simulink model "ABLS_Model"  (R2025a)
settings: Solver=FixedStepDiscrete  StartTime=0.0  StopTime=10.0  FixedStep=0.01  RelTol=1e-3
undefined symbols (not defined in the file): dspblkCoreblockFVToolHelper, gcbh, Ts
libraries: simulink x3
settings Model: Creator=Gagan  LastModifiedBy=Gagan

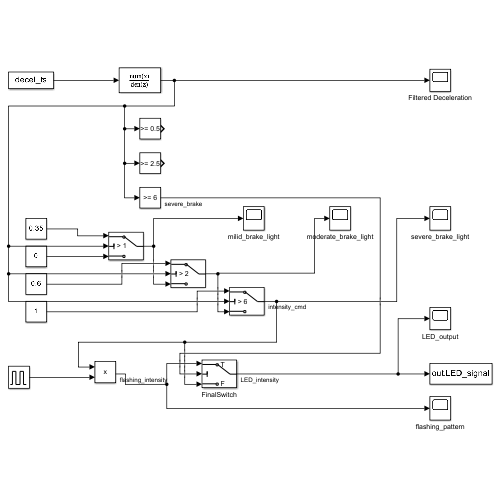
[thumbnail: Simulink's stored preview of the top-level diagram]
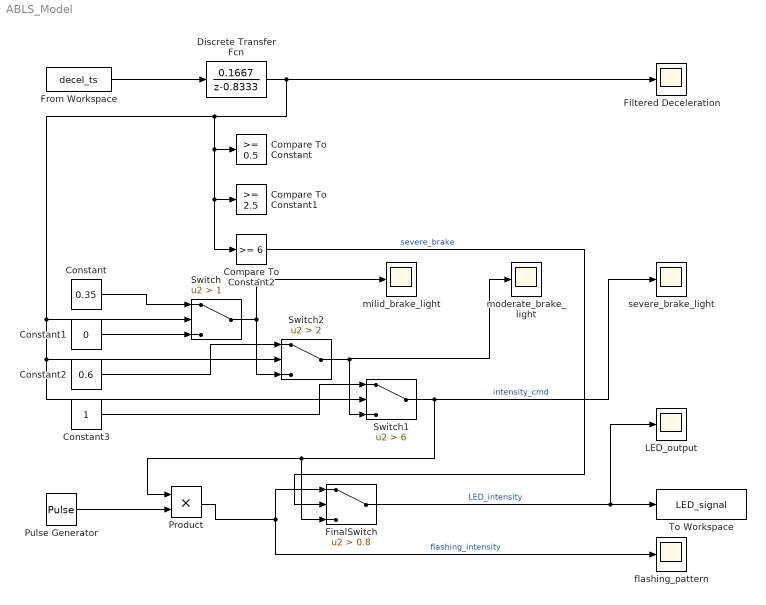
== system ABLS_Model ==
  Compare To Constant : simulink/Logic and Bit Operations/Compare To Constant  relop=>=  const=0.5  OutDataTypeStr=boolean
  Compare To Constant1 : simulink/Logic and Bit Operations/Compare To Constant  relop=>=  const=2.5  OutDataTypeStr=boolean
  Compare To Constant2 : simulink/Logic and Bit Operations/Compare To Constant  relop=>=  const=6  OutDataTypeStr=boolean
  Constant : Constant  Value=0.35
  Constant1 : Constant  Value=0
  Constant2 : Constant  Value=0.6
  Constant3 : Constant
  Discrete Transfer Fcn : DiscreteTransferFcn  LoadFcn=dspblkCoreblockFVToolHelper(gcbh,'load');  Numerator=[0.1667]  Denominator=[1 -0.8333]
      settings: CopyFcn=dspblkCoreblockFVToolHelper(gcbh,'copy');  DeleteFcn=dspblkCoreblockFVToolHelper(gcbh,'close');  ModelCloseFcn=dspblkCoreblockFVToolHelper(gcbh,'close');  PreSaveFcn=dspblkCoreblockFVToolHelper(gcbh,'presave');  PostSaveFcn=dspblkCoreblockFVToolHelper(gcbh,'postsave');  CloseFcn=dspblkCoreblockFVToolHelper(gcbh,'close');
  Filtered Deceleration : Scope
      settings: ActiveDisplayYMinimum=-2.4650997941637955  ActiveDisplayYMaximum=10.638541253611827
  FinalSwitch : Switch  Criteria=u2 > Threshold  Threshold=0.8  SaturateOnIntegerOverflow=off  InputSameDT=off
  From Workspace : FromWorkspace  VariableName=decel_ts  SampleTime=Ts
  LED_output : Scope
      settings: ActiveDisplayYMinimum=-0.43818211728905965  ActiveDisplayYMaximum=1.4045280690428719
  Product : Product
  Pulse Generator : DiscretePulseGenerator  PulseType=Time based  Period=0.2  PulseWidth=50
  Switch : Switch  Criteria=u2 > Threshold  Threshold=1  SaturateOnIntegerOverflow=off  InputSameDT=off
  Switch1 : Switch  Criteria=u2 > Threshold  Threshold=6  SaturateOnIntegerOverflow=off  InputSameDT=off
  Switch2 : Switch  Criteria=u2 > Threshold  Threshold=2  SaturateOnIntegerOverflow=off  InputSameDT=off
  To Workspace : ToWorkspace  VariableName=LED_signal  SaveFormat=Timeseries  SampleTime=0.01
  flashing_pattern : Scope
      settings: ActiveDisplayYMinimum=-0.86657175559493416  ActiveDisplayYMaximum=1.29697667869826  DataLoggingVariableName=ScopeData7
  milid_brake_light : Scope
      settings: ActiveDisplayYMinimum=-0.0913088843903277  ActiveDisplayYMaximum=0.78387268310085778  DataLoggingVariableName=ScopeData2
  moderate_brake_light : Scope
      settings: ActiveDisplayYMinimum=-1.3463811582378364  ActiveDisplayYMaximum=1.7268034889270079  DataLoggingVariableName=ScopeData4
  severe_brake_light : Scope
      settings: ActiveDisplayYMinimum=-0.38415240970724662  ActiveDisplayYMaximum=1.4741521320498872  DataLoggingVariableName=ScopeData5
  wires:
  Discrete Transfer Fcn/1 -> Switch/2, Switch1/2, Switch2/2, Compare To Constant2/1, Compare To Constant1/1, Compare To Constant/1, Filtered Deceleration/1
  Constant/1 -> Switch/1
  Constant1/1 -> Switch/3
  Switch/1 -> Switch2/3, milid_brake_light/1
  Constant2/1 -> Switch2/1
  Switch2/1 -> Switch1/3, moderate_brake_light/1
  Constant3/1 -> Switch1/1
  Switch1/1 -> severe_brake_light/1, FinalSwitch/3, Product/1  "intensity_cmd"
  Compare To Constant2/1 -> FinalSwitch/2  "severe_brake"
  Product/1 -> FinalSwitch/1, flashing_pattern/1  "flashing_intensity"
  FinalSwitch/1 -> LED_output/1, To Workspace/1  "LED_intensity"
  From Workspace/1 -> Discrete Transfer Fcn/1
  Pulse Generator/1 -> Product/2
